simulink model "refuel_model"  (R2021b)
settings: Solver=ode15s  StartTime=0.0  StopTime=tsim  MinStep=min_step  RelTol=1e-3  EnableMultiTasking=on
InitFcn:
  | min_step=1e-12;
  | warning 'off';
values from neighbouring files (symbols this model uses):
  area_valve = (pi*dpipe^2/4)    (= 4.90166993776e-05)    [script_compressor.m]    (also in script_refuel.m)
  ki = 0.01/1e3    (= 1e-05)    [script_refuel.m]
  ki_cool = 1e4    (= 10000)    [script_refuel.m]
  Kmin = 0.05    [script_H2_assumption.m]    (also in script_refuel.m = 0.00125)
  kp = 0.01    [script_refuel.m]
  kp_cool = 1e4    (= 10000)    [script_refuel.m]
  Kv1 = 1    [script_H2_assumption.m]    (also in script_compressor.m = 0.025; script_refuel.m = 0.025)
  Kv2 = Kv1    (= 1)    [script_H2_assumption.m]    (also in script_refuel.m = 0.025)
  ph2_rate = 100/60    (= 1.66666666667)    [script_compressor.m]    (also in script_refuel.m)
  R_h2 = 4.12    [script_H2_assumption.m]    (also in script_compressor.m; script_init_pressures.m; script_pipe_dim.m; script_refuel.m)
  tc = 1000    [script_H2_assumption.m]    (also in script_refuel.m)
  tsim = 2000    [script_H2_assumption.m]    (also in script_compressor.m; script_init_pressures.m = 10; script_pipe_dim.m = 30; script_refuel.m)
  vch_o = 0.125    [script_compressor.m]    (also in script_init_pressures.m; script_pipe_dim.m; script_refuel.m)
libraries: fl_lib x36, nesl_utility x7, slpidlib x2, simulink x1
(part 1 of 4)
settings Model: Creator=jsagardu  LastModifiedBy=jsagardu
settings SolverCC: InitialStep=min_step  AlgebraicLoopSolver=TrustRegion
settings DataIOCC: ReturnWorkspaceOutputs=off
settings OptimizationCC: LifeSpan=inf
settings DebuggingCC: SFUnexpectedBacktrackingDiag=warning  SFNoUnconditionalDefaultTransitionDiag=warning  SFExecutionAtInitializationDiag=none  SFMachineParentedDataDiag=warning  ArithmeticOperatorsInVariantConditions=warning
settings SFSimCC: SimUseLocalCustomCode=off  CustomCodeUndefinedFunction=UseInterfaceOnly
settings RTWCC: RTWUseLocalCustomCode=off
settings CodeAppCC: StateflowObjectComments=on
settings GRTTargetCC: TargetLangStandard=C89/C90 (ANSI)
settings ConfigComp: CovMetricSettings=dw  CovSaveCumulativeToWorkspaceVar=on  CovSaveSingleToWorkspaceVar=on  CovExternalEMLEnable=off
settings SimscapeCC: SimscapeNormalizeSystem=off  SimscapeLogType=local  SimscapeLogLimitData=off  SimscapeLogDataHistory=10000

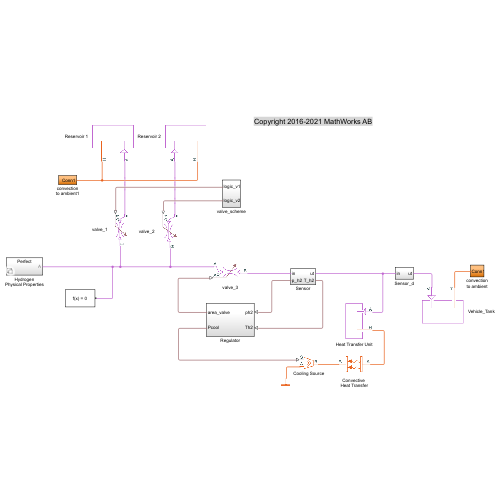
[thumbnail: Simulink's stored preview of the top-level diagram]
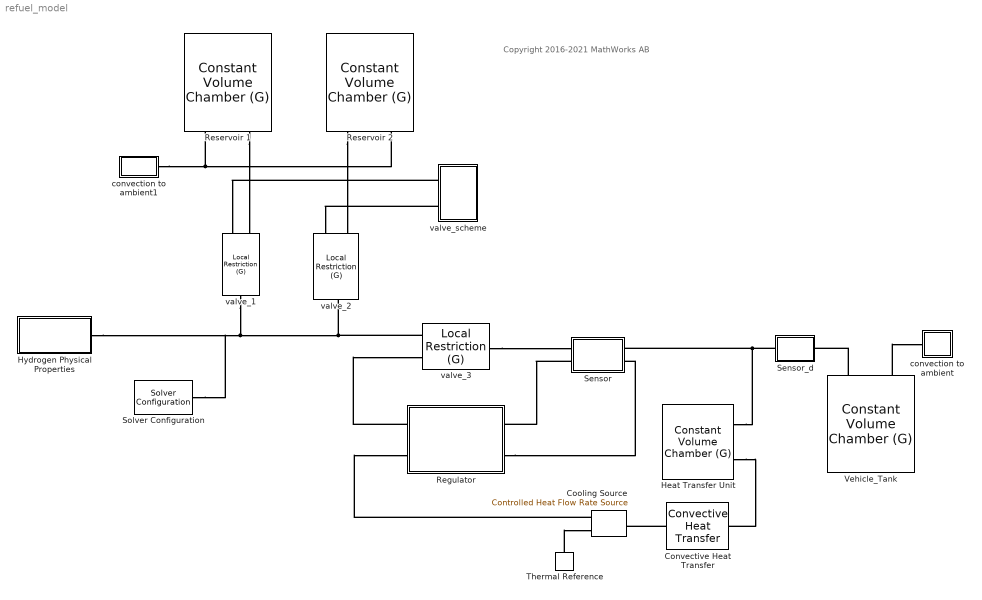
== system refuel_model ==
  note: Copyright 2016-2021 MathWorks AB
  Convective Heat Transfer : fl_lib/Thermal/Thermal Elements/Convective Heat Transfer  area=area_ht m^2  heat_tr_coeff=alpha_ht W/(m^2 * K)  T_specify=off  T_priority=None  T=0 K  T_nominal_specify=off  T_nominal_unit=K  T_nominal_value=1  Q_specify=off  Q_priority=None  Q=0 J/s  Q_nominal_specify=off  Q_nominal_unit=W  Q_nominal_value=1
  Cooling Source : fl_lib/Thermal/Thermal Sources/Controlled Heat Flow Rate Source
      settings: LogSimulationData=on
  Heat Transfer Unit : fl_lib/Gas/Elements/Constant Volume Chamber (G)  volume=vol_ht m^3  num_ports=foundation.enum.num_ports.one  area_A=0.01 m^2  area_B=0.01 m^2  area_C=0.01 m^2  area_D=0.01 m^2  p_I_specify=on  p_I_priority=High  p_I=po_init bar  p_I_nominal_specify=off  p_I_nominal_unit=MPa  p_I_nominal_value=1  T_I_specify=on  T_I_priority=High  T_I=To_init K  T_I_nominal_specify=off  T_I_nominal_unit=K  T_I_nominal_value=1  rho_chamber_specify=off  rho_chamber_priority=None  rho_chamber=1.2 kg/m^3  rho_chamber_nominal_specify=off  rho_chamber_nominal_unit=kg/m^3  rho_chamber_nominal_value=1
      settings: SourceProductBaseCode=SS  LogSimulationData=on  InternalSimscapePortConfiguration="{\"Bottom\":[],\"Left\":[{\"id\":\"A\",\"label\":\"A\",\"type\":\"foundation.gas.gas\"},{\"id\":\"H\",\"label\":\"H\",\"type\":\"foundation.thermal.thermal\"}],\"Right\":[],\"Top\":[]}"
  Hydrogen Physical Properties : Subsystem  Variant=on
  Regulator : Subsystem
  Reservoir 1 : fl_lib/Gas/Elements/Constant Volume Chamber (G)  volume=vch_i1 m^3  num_ports=foundation.enum.num_ports.one  area_A=0.01 m^2  area_B=0.01 m^2  area_C=0.01 m^2  area_D=0.01 m^2  p_I_specify=on  p_I_priority=High  p_I=pi1_init bar  p_I_nominal_specify=off  p_I_nominal_unit=MPa  p_I_nominal_value=1  T_I_specify=on  T_I_priority=High  T_I=Ti_init K  T_I_nominal_specify=off  T_I_nominal_unit=K  T_I_nominal_value=1  rho_chamber_specify=off  rho_chamber_priority=None  rho_chamber=1.2 kg/m^3  rho_chamber_nominal_specify=off  rho_chamber_nominal_unit=kg/m^3  rho_chamber_nominal_value=1
      settings: SourceProductBaseCode=SS  InternalSimscapePortConfiguration="{\"Bottom\":[],\"Left\":[{\"id\":\"A\",\"label\":\"A\",\"type\":\"foundation.gas.gas\"},{\"id\":\"H\",\"label\":\"H\",\"type\":\"foundation.thermal.thermal\"}],\"Right\":[],\"Top\":[]}"
  Reservoir 2 : fl_lib/Gas/Elements/Constant Volume Chamber (G)  volume=vch_i2 m^3  num_ports=foundation.enum.num_ports.one  area_A=0.01 m^2  area_B=0.01 m^2  area_C=0.01 m^2  area_D=0.01 m^2  p_I_specify=on  p_I_priority=High  p_I=pi2_init bar  p_I_nominal_specify=off  p_I_nominal_unit=MPa  p_I_nominal_value=1  T_I_specify=on  T_I_priority=High  T_I=Ti_init K  T_I_nominal_specify=off  T_I_nominal_unit=K  T_I_nominal_value=1  rho_chamber_specify=off  rho_chamber_priority=None  rho_chamber=1.2 kg/m^3  rho_chamber_nominal_specify=off  rho_chamber_nominal_unit=kg/m^3  rho_chamber_nominal_value=1
      settings: SourceProductBaseCode=SS  InternalSimscapePortConfiguration="{\"Bottom\":[],\"Left\":[{\"id\":\"A\",\"label\":\"A\",\"type\":\"foundation.gas.gas\"},{\"id\":\"H\",\"label\":\"H\",\"type\":\"foundation.thermal.thermal\"}],\"Right\":[],\"Top\":[]}"
  Sensor : Subsystem
  Sensor_d : Subsystem
  Solver Configuration : nesl_utility/Solver Configuration  PhysicalDomain=network_engine_domain  SubClassName=solver  LeftPortType=input  RightPortType=generic  Tones=[]  Harmonics=[]  SimulateNoise=off  Profile=off  UseLocalSampling=off  EnableSwitchedLinearOptims=on  FrequencyDomain=off  UseCCode=off  RelTol=0.001  AbsTol=1e-06  MinStep=1e-09  ToWorkspace=off  RevertToSquareIcSolve=off  NumHomotopyIterations=100  PhasorMode=off  PhasorModeNumHarmonics=1  DoDC=off  ResidualTolerance=1e-09  UseLocalSolver=on  LocalSolverChoice=NE_BACKWARD_EULER_ADVANCER  LocalSolverSampleTime=0.1  DoFixedCost=on  MaxNonlinIter=3  MaxModeIter=2  ComputeImpulses=off  ImpulseIterations=2  LinearAlgebra=Sparse  EquationFormulation=NE_TIME_EF  DelaysMemoryBudget=1024  AutomaticFiltering=on  FilteringTimeConstant=0.001  PartitionStorageMethod=AS_NEEDED  PartitionMemoryBudget=1024  PartitionMethod=FAST
      settings: SourceProductBaseCode=PW,SS
  Thermal Reference : fl_lib/Thermal/Thermal Elements/Thermal Reference
  Vehicle_Tank : fl_lib/Gas/Elements/Constant Volume Chamber (G)  volume=vch_o m^3  num_ports=foundation.enum.num_ports.one  area_A=0.01 m^2  area_B=0.01 m^2  area_C=0.01 m^2  area_D=0.01 m^2  p_I_specify=on  p_I_priority=High  p_I=po_init bar  p_I_nominal_specify=off  p_I_nominal_unit=MPa  p_I_nominal_value=1  T_I_specify=on  T_I_priority=High  T_I=To_init K  T_I_nominal_specify=off  T_I_nominal_unit=K  T_I_nominal_value=1  rho_chamber_specify=off  rho_chamber_priority=None  rho_chamber=1.2 kg/m^3  rho_chamber_nominal_specify=off  rho_chamber_nominal_unit=kg/m^3  rho_chamber_nominal_value=1
      settings: SourceProductBaseCode=SS  LogSimulationData=on  InternalSimscapePortConfiguration="{\"Bottom\":[],\"Left\":[{\"id\":\"A\",\"label\":\"A\",\"type\":\"foundation.gas.gas\"},{\"id\":\"H\",\"label\":\"H\",\"type\":\"foundation.thermal.thermal\"}],\"Right\":[],\"Top\":[]}"
  convection to ambient : Subsystem
  convection to ambient1 : Subsystem
  valve_1 : fl_lib/Gas/Elements/Local Restriction (G)  restriction_type=foundation.enum.restriction_type.variable  restriction_area=1e-3 m^2  min_area=Kmin*area_valve m^2  max_area=0.005 m^2  area=0.01 m^2  Cd=0.82  B_lam=0.999
      settings: SourceProductBaseCode=SS  InternalSimscapePortConfiguration="{\"Bottom\":[],\"Left\":[{\"id\":\"A\",\"label\":\"A\",\"type\":\"foundation.gas.gas\"},{\"id\":\"area_in\",\"label\":\"AR\",\"type\":\"input\"}],\"Right\":[{\"id\":\"B\",\"label\":\"B\",\"type\":\"foundation.gas.gas\"}],\"Top\":[]}"
  valve_2 : fl_lib/Gas/Elements/Local Restriction (G)  restriction_type=foundation.enum.restriction_type.variable  restriction_area=1e-3 m^2  min_area=Kmin*area_valve m^2  max_area=0.005 m^2  area=0.01 m^2  Cd=0.82  B_lam=0.999
      settings: SourceProductBaseCode=SS  LogSimulationData=on  InternalSimscapePortConfiguration="{\"Bottom\":[],\"Left\":[{\"id\":\"A\",\"label\":\"A\",\"type\":\"foundation.gas.gas\"},{\"id\":\"area_in\",\"label\":\"AR\",\"type\":\"input\"}],\"Right\":[{\"id\":\"B\",\"label\":\"B\",\"type\":\"foundation.gas.gas\"}],\"Top\":[]}"
  valve_3 : fl_lib/Gas/Elements/Local Restriction (G)  restriction_type=foundation.enum.restriction_type.variable  restriction_area=1e-3 m^2  min_area=1e-12 m^2  max_area=0.005 m^2  area=0.01 m^2  Cd=0.82  B_lam=0.999
      settings: SourceProductBaseCode=SS  LogSimulationData=on  InternalSimscapePortConfiguration="{\"Bottom\":[],\"Left\":[{\"id\":\"A\",\"label\":\"A\",\"type\":\"foundation.gas.gas\"},{\"id\":\"area_in\",\"label\":\"AR\",\"type\":\"input\"}],\"Right\":[{\"id\":\"B\",\"label\":\"B\",\"type\":\"foundation.gas.gas\"}],\"Top\":[]}"
  valve_scheme : Subsystem
  connections:
  valve_3/RConn1 -- Sensor/LConn1
  convection to ambient1/LConn1 -- Reservoir 2/LConn2 -- Reservoir 1/LConn2
  Sensor/LConn2 -- Regulator/RConn1
  Sensor_d/LConn1 -- Sensor/RConn1 -- Heat Transfer Unit/LConn1
  Regulator/RConn2 -- Sensor/RConn2
  Thermal Reference/LConn1 -- Cooling Source/RConn2
  Convective Heat Transfer/RConn1 -- Cooling Source/LConn1
  Heat Transfer Unit/LConn2 -- Convective Heat Transfer/LConn1
  Vehicle_Tank/LConn1 -- Sensor_d/RConn1
  Vehicle_Tank/LConn2 -- convection to ambient/LConn1
  valve_3/LConn1 -- Hydrogen Physical Properties/RConn1 -- Solver Configuration/RConn1 -- valve_1/RConn1 -- valve_2/RConn1
  Reservoir 1/LConn1 -- valve_1/LConn1
  Reservoir 2/LConn1 -- valve_2/LConn1
  valve_scheme/LConn2 -- valve_2/LConn2
  Regulator/LConn1 -- valve_3/LConn2
  Cooling Source/RConn1 -- Regulator/LConn2
  valve_scheme/LConn1 -- valve_1/LConn2

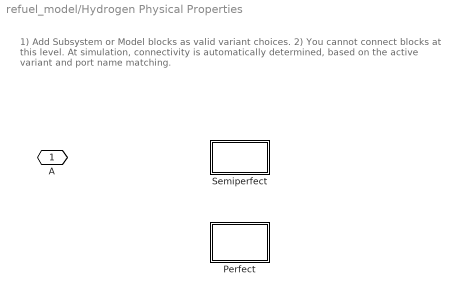
== system refuel_model/Hydrogen Physical Properties ==
  note: 1) Add Subsystem or Model blocks as valid variant choices.
      | 2) You cannot connect blocks at this level. At simulation, connectivity is automatically
      | determined, based on the active variant and port name matching.
  Perfect : Subsystem  VariantControl=var_a>0
  Semiperfect : Subsystem  VariantControl=var_b>0
  A : PMIOPort  Side=Right

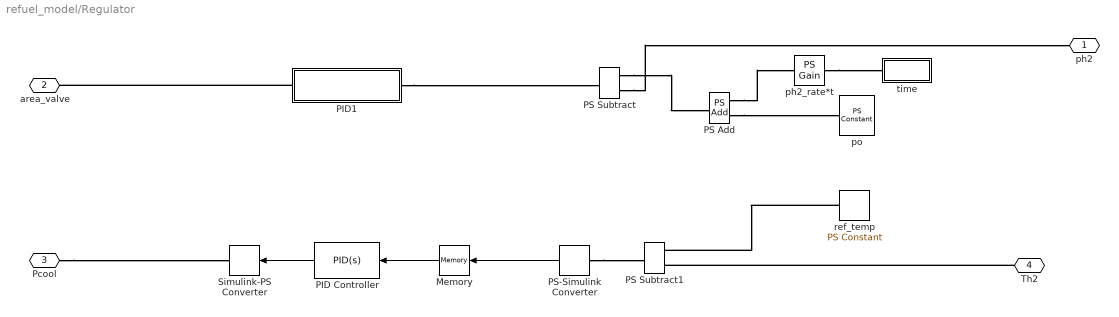
== system refuel_model/Regulator ==
  Memory : Memory
  PID Controller : slpidlib/PID Controller  Controller=PID  Form=Parallel  TimeDomain=Continuous-time  UseExternalTs=off  SampleTime=-1  IntegratorMethod=Forward Euler  FilterMethod=Forward Euler  ControllerParametersSource=internal  P=kp_cool  I=ki_cool  D=0  UseFilter=on  N=100  TunerSelectOption=Transfer Function Based (PID Tuner App)  InitialConditionSource=internal  InitialConditionForIntegrator=0  InitialConditionForFilter=0  DifferentiatorICPrevScaledInput=0  ExternalReset=none  TrackingMode=off  Kt=1  LimitOutput=on  SatLimitsSource=internal  UpperSaturationLimit=1e5  LowerSaturationLimit=-1e5  LinearizeAsGain=on  AntiWindupMode=back-calculation  Kb=100  POutMin=[]  POutMax=[]  IOutMin=[]  IOutMax=[]  DOutMin=[]  DOutMax=[]  NOutMin=[]  NOutMax=[]  SumOutMin=[]  SumOutMax=[]  SaturationOutMin=[]  SaturationOutMax=[]  PParamMin=[]  PParamMax=[]  IParamMin=[]  IParamMax=[]  DParamMin=[]  DParamMax=[]  NParamMin=[]  NParamMax=[]  KbParamMin=[]  KbParamMax=[]  KtParamMin=[]  KtParamMax=[]  KbOutMin=[]  KbOutMax=[]  KtOutMin=[]  KtOutMax=[]  IntegratorOutMin=[]  IntegratorOutMax=[]  FilterOutMin=[]  FilterOutMax=[]  SumI1OutMin=[]  SumI1OutMax=[]  SumI2OutMin=[]  SumI2OutMax=[]  SumI3OutMin=[]  SumI3OutMax=[]  SumI4OutMin=[]  SumI4OutMax=[]  SumDOutMin=[]  SumDOutMax=[]  DifferentiatorOutMin=[]  DifferentiatorOutMax=[]  FilterDiffOutCoefMin=[]  FilterDiffOutCoefMax=[]  ReciprocalOutMin=[]  ReciprocalOutMax=[]  SumDenOutMin=[]  SumDenOutMax=[]  SumNumOutMin=[]  SumNumOutMax=[]  DivideOutMin=[]  DivideOutMax=[]  UdiffTsProdOutMin=[]  UdiffTsProdOutMax=[]  NTsProdOutMin=[]  NTsProdOutMax=[]  UintegralTsProdOutMin=[]  UintegralTsProdOutMax=[]  UngainTsProdOutMin=[]  UngainTsProdOutMax=[]  IntegratorContinuousStateAttributes=''  IntegratorStateMustResolveToSignalObject=off  IntegratorRTWStateStorageClass=Auto  FilterContinuousStateAttributes=''  FilterStateMustResolveToSignalObject=off  FilterRTWStateStorageClass=Auto  ParallelPVariant=InternalParameters  IdealPVariant=Disabled  IVariant=InternalParameters  DVariant=InternalParameters  IntegratorVariant=Continuous  SatVariant=Enabled  AWVariant=BackCalculation  PCopyVariant=Disabled  TRVariant=Disabled  FdbkBlocksVariant=Forward  IdealPFdbkVariant=Disabled  SatFdbkVariant=Disabled  DerivativeFilterVariant=ContFilter  NVariant=InternalParameters  NCopyVariant=Disabled  FilterICVariant=InternalICsFilter  IntegratorICVariant=InternalICs  ExternalResetVariant=Disabled  TRSumVariant=Passthrough  SumFdbkVariant=Disabled  SumVariant=Sum_PID  TsampFilterVariant=InternalTs  TsampNgainVariant=Passthrough  TsampIntegralVariant=Passthrough  ExternalSaturationOutDataTypeStr=Inherit: Same as second input
  PID1 : Subsystem
  PS Add : fl_lib/Physical Signals/Functions/PS Add
  PS Subtract : fl_lib/Physical Signals/Functions/PS Subtract
  PS Subtract1 : fl_lib/Physical Signals/Functions/PS Subtract
  PS-Simulink Converter : nesl_utility/PS-Simulink Converter  PhysicalDomain=network_engine_domain  SubClassName=ps_output  LeftPortType=input  RightPortType=output  PseudoPeriodic=off  Frequencies=[]  Unit=K  AffineConversion=off
      settings: SourceProductBaseCode=PW,SS
  Simulink-PS Converter : nesl_utility/Simulink-PS Converter  PhysicalDomain=network_engine_domain  SubClassName=ps_input  LeftPortType=input  RightPortType=output  PseudoPeriodic=off  Frequencies=[]  NoiseDistribution=none  NoiseParameters=[]  Unit=1  AffineConversion=off  FilteringAndDerivatives=zero  SimscapeFilterOrder=1  InputFilterTimeConstant=0.001  UdotUserProvided=1
      settings: SourceProductBaseCode=PW,SS
  ph2_rate*t : fl_lib/Physical Signals/Functions/PS Gain  gain=ph2_rate bar/s
  po : fl_lib/Physical Signals/Sources/PS Constant  constant=po_init bar
  ref_temp : fl_lib/Physical Signals/Sources/PS Constant  constant=Th2_ref K
  time : Subsystem
  ph2 : PMIOPort  Side=Right
  area_valve : PMIOPort  Port=2  Side=Left
  Pcool : PMIOPort  Port=3  Side=Left
  Th2 : PMIOPort  Port=4  Side=Right
  wires:
  PID Controller/1 -> Simulink-PS Converter/1
  PS-Simulink Converter/1 -> Memory/1
  Memory/1 -> PID Controller/1
  connections:
  PS Subtract/LConn1 -- PS Add/RConn1
  ph2_rate*t/LConn1 -- time/LConn1
  PS Add/LConn1 -- ph2_rate*t/RConn1
  PS Add/LConn2 -- po/RConn1
  PS Subtract/LConn2 -- ph2/RConn1
  PS-Simulink Converter/LConn1 -- PS Subtract1/RConn1
  Pcool/RConn1 -- Simulink-PS Converter/RConn1
  Th2/RConn1 -- PS Subtract1/LConn2
  PID1/RConn1 -- PS Subtract/RConn1
  PID1/LConn1 -- area_valve/RConn1
  ref_temp/RConn1 -- PS Subtract1/LConn1

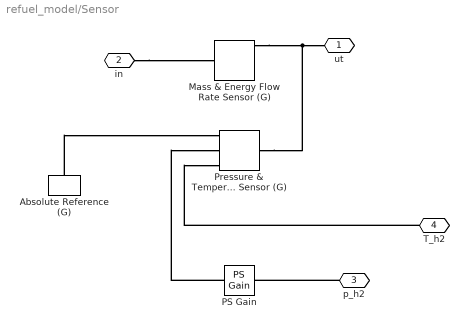
== system refuel_model/Sensor ==
  Absolute Reference (G) : fl_lib/Gas/Elements/Absolute Reference (G)
      settings: SourceProductBaseCode=SS  InternalSimscapePortConfiguration="{\"Bottom\":[],\"Left\":[{\"id\":\"A\",\"label\":\"\",\"type\":\"foundation.gas.gas\"}],\"Right\":[],\"Top\":[]}"
  Mass & Energy Flow Rate Sensor (G) : fl_lib/Gas/Sensors/Mass & Energy Flow Rate Sensor (G)
      settings: SourceProductBaseCode=SS  InternalSimscapePortConfiguration="{\"Bottom\":[],\"Left\":[{\"id\":\"A\",\"label\":\"A\",\"type\":\"foundation.gas.gas\"}],\"Right\":[{\"id\":\"B\",\"label\":\"B\",\"type\":\"foundation.gas.gas\"},{\"id\":\"M\",\"label\":\"M\",\"type\":\"output\"},{\"id\":\"PHI\",\"label\":\"Phi\",\"type\":\"output\"}],\"Top\":[]}"
  PS Gain : fl_lib/Physical Signals/Functions/PS Gain  gain=1/1e5 bar/Pa
  Pressure & Temperature Sensor (G) : fl_lib/Gas/Sensors/Pressure & Temperature Sensor (G)
      settings: SourceProductBaseCode=SS  LogSimulationData=on  InternalSimscapePortConfiguration="{\"Bottom\":[],\"Left\":[{\"id\":\"A\",\"label\":\"A\",\"type\":\"foundation.gas.gas\"}],\"Right\":[{\"id\":\"B\",\"label\":\"B\",\"type\":\"foundation.gas.gas\"},{\"id\":\"P\",\"label\":\"P\",\"type\":\"output\"},{\"id\":\"T\",\"label\":\"T\",\"type\":\"output\"}],\"Top\":[]}"
  ut : PMIOPort  Side=Right
  in : PMIOPort  Port=2  Side=Left
  p_h2 : PMIOPort  Port=3  Side=Left
  T_h2 : PMIOPort  Port=4  Side=Right
  connections:
  p_h2/RConn1 -- PS Gain/RConn1
  PS Gain/LConn1 -- Pressure & Temperature Sensor (G)/RConn2
  Absolute Reference (G)/LConn1 -- Pressure & Temperature Sensor (G)/RConn1
  in/RConn1 -- Mass & Energy Flow Rate Sensor (G)/LConn1
  Mass & Energy Flow Rate Sensor (G)/RConn1 -- Pressure & Temperature Sensor (G)/LConn1 -- ut/RConn1
  T_h2/RConn1 -- Pressure & Temperature Sensor (G)/RConn3

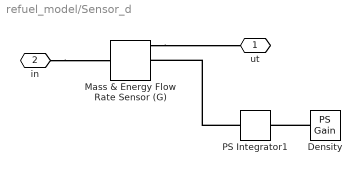
== system refuel_model/Sensor_d ==
  Density : fl_lib/Physical Signals/Functions/PS Gain  gain=1/vch_o kg/m^3
      settings: LogSimulationData=on
  Mass & Energy Flow Rate Sensor (G) : fl_lib/Gas/Sensors/Mass & Energy Flow Rate Sensor (G)
      settings: SourceProductBaseCode=SS  InternalSimscapePortConfiguration="{\"Bottom\":[],\"Left\":[{\"id\":\"A\",\"label\":\"A\",\"type\":\"foundation.gas.gas\"}],\"Right\":[{\"id\":\"B\",\"label\":\"B\",\"type\":\"foundation.gas.gas\"},{\"id\":\"M\",\"label\":\"M\",\"type\":\"output\"},{\"id\":\"PHI\",\"label\":\"Phi\",\"type\":\"output\"}],\"Top\":[]}"
  PS Integrator1 : fl_lib/Physical Signals/Linear Operators/PS Integrator  reset_method=foundation.enum.IntegratorResetSpec.None  initial_condition_spec=foundation.enum.IntegratorICSpec.Internal  x0=0 kg
      settings: SourceProductBaseCode=SS
  ut : PMIOPort  Side=Right
  in : PMIOPort  Port=2  Side=Left
  connections:
  Mass & Energy Flow Rate Sensor (G)/RConn1 -- ut/RConn1
  in/RConn1 -- Mass & Energy Flow Rate Sensor (G)/LConn1
  PS Integrator1/LConn1 -- Mass & Energy Flow Rate Sensor (G)/RConn2
  Density/LConn1 -- PS Integrator1/RConn1

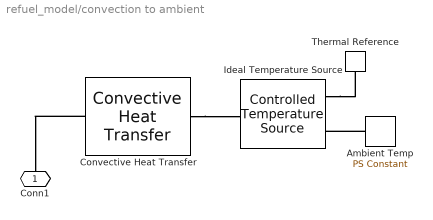
== system refuel_model/convection to ambient ==
  Ambient Temp : fl_lib/Physical Signals/Sources/PS Constant  constant=Tamb
  Convective Heat Transfer : fl_lib/Thermal/Thermal Elements/Convective Heat Transfer  area=1e-4 m^2  heat_tr_coeff=alpha W/(m^2 * K)  T_specify=off  T_priority=None  T=0 K  T_nominal_specify=off  T_nominal_unit=K  T_nominal_value=1  Q_specify=off  Q_priority=None  Q=0 J/s  Q_nominal_specify=off  Q_nominal_unit=W  Q_nominal_value=1
  Ideal Temperature Source : fl_lib/Thermal/Thermal Sources/Controlled Temperature Source
  Thermal Reference : fl_lib/Thermal/Thermal Elements/Thermal Reference
  Conn1 : PMIOPort  Side=Left
  connections:
  Ambient Temp/RConn1 -- Ideal Temperature Source/RConn1
  Ideal Temperature Source/RConn2 -- Thermal Reference/LConn1
  Convective Heat Transfer/LConn1 -- Conn1/RConn1
  Convective Heat Transfer/RConn1 -- Ideal Temperature Source/LConn1

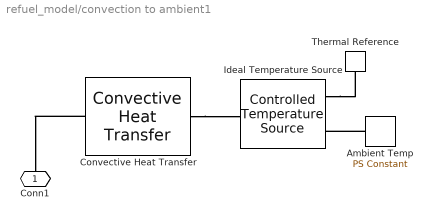
== system refuel_model/convection to ambient1 ==
  Ambient Temp : fl_lib/Physical Signals/Sources/PS Constant  constant=Tamb
  Convective Heat Transfer : fl_lib/Thermal/Thermal Elements/Convective Heat Transfer  area=1e-4 m^2  heat_tr_coeff=alpha W/(m^2 * K)  T_specify=off  T_priority=None  T=0 K  T_nominal_specify=off  T_nominal_unit=K  T_nominal_value=1  Q_specify=off  Q_priority=None  Q=0 J/s  Q_nominal_specify=off  Q_nominal_unit=W  Q_nominal_value=1
  Ideal Temperature Source : fl_lib/Thermal/Thermal Sources/Controlled Temperature Source
  Thermal Reference : fl_lib/Thermal/Thermal Elements/Thermal Reference
  Conn1 : PMIOPort  Side=Left
  connections:
  Ambient Temp/RConn1 -- Ideal Temperature Source/RConn1
  Ideal Temperature Source/RConn2 -- Thermal Reference/LConn1
  Convective Heat Transfer/LConn1 -- Conn1/RConn1
  Convective Heat Transfer/RConn1 -- Ideal Temperature Source/LConn1

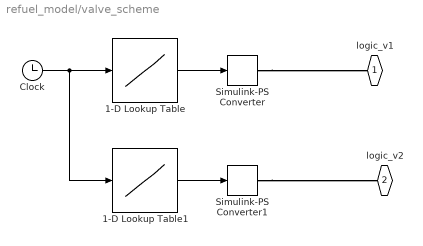
== system refuel_model/valve_scheme ==
  1-D Lookup Table : Lookup_n-D  NumberOfTableDimensions=1  BreakpointsForDimension1=[0 tc tc+0.1 tsim]  Table=[Kv1 Kv1 0 0]*area_valve  InternalRulePriority=Speed  RndMeth=Simplest  InputSameDT=on
  1-D Lookup Table1 : Lookup_n-D  NumberOfTableDimensions=1  BreakpointsForDimension1=[0 tc tc+0.1 tsim]  Table=[0 0 Kv2 Kv2]*area_valve  InternalRulePriority=Speed  RndMeth=Simplest  InputSameDT=on
  Clock : Clock
  Simulink-PS Converter : nesl_utility/Simulink-PS Converter  PhysicalDomain=network_engine_domain  SubClassName=ps_input  LeftPortType=input  RightPortType=output  PseudoPeriodic=off  Frequencies=[]  NoiseDistribution=none  NoiseParameters=[]  Unit=1  AffineConversion=off  FilteringAndDerivatives=filter  SimscapeFilterOrder=1  InputFilterTimeConstant=tf  UdotUserProvided=1
      settings: SourceProductBaseCode=PW,SS
  Simulink-PS Converter1 : nesl_utility/Simulink-PS Converter  PhysicalDomain=network_engine_domain  SubClassName=ps_input  LeftPortType=input  RightPortType=output  PseudoPeriodic=off  Frequencies=[]  NoiseDistribution=none  NoiseParameters=[]  Unit=1  AffineConversion=off  FilteringAndDerivatives=filter  SimscapeFilterOrder=1  InputFilterTimeConstant=tf  UdotUserProvided=1
      settings: SourceProductBaseCode=PW,SS
  logic_v1 : PMIOPort  Side=Left
  logic_v2 : PMIOPort  Port=2  Side=Left
  wires:
  Clock/1 -> 1-D Lookup Table1/1, 1-D Lookup Table/1
  1-D Lookup Table1/1 -> Simulink-PS Converter1/1
  1-D Lookup Table/1 -> Simulink-PS Converter/1
  connections:
  Simulink-PS Converter1/RConn1 -- logic_v2/RConn1
  Simulink-PS Converter/RConn1 -- logic_v1/RConn1
